simulink model "task_2_sim"  (R2023a)
settings: Solver=VariableStepAuto  StartTime=0.0  StopTime=15  MaxStep=1e-4  RelTol=1e-4
undefined symbols (not defined in the file): A_b, B_b, C_b, D, G, G_g, iQ, K, Kf, Kg, L, w_g0, wfx_0, Y, Y_g
settings Model: Creator=user  LastModifiedBy=user

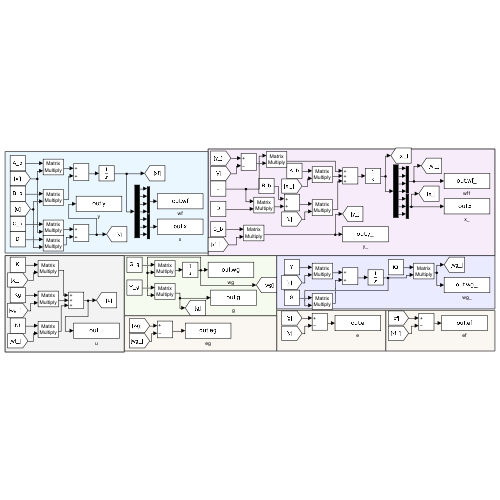
[thumbnail: Simulink's stored preview of the top-level diagram]
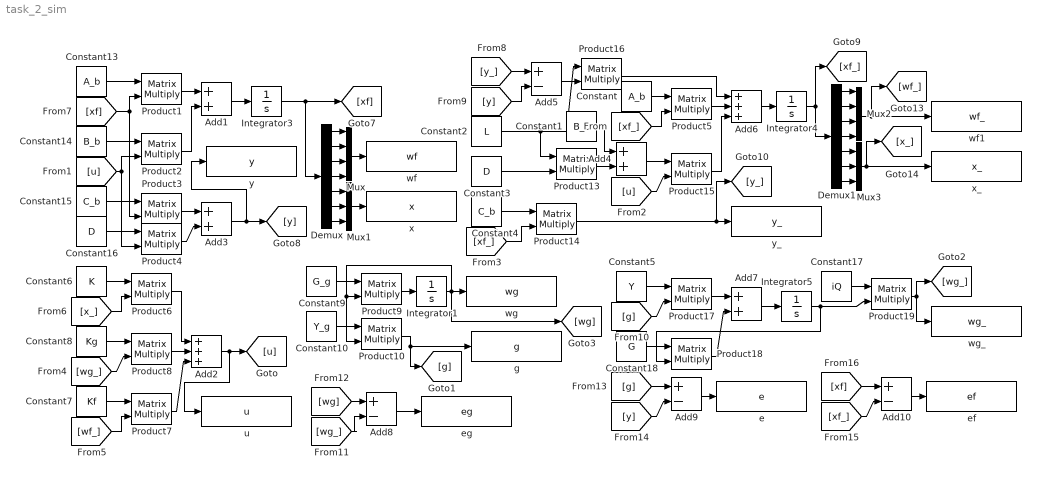
== system task_2_sim ==
  Add{1,3..4,7} (4 alike) : Sum
  Add{5,8..10} (4 alike) : Sum  Inputs=+-
  Add2 : Sum  Inputs=+++
  Add6 : Sum  Inputs=+++
  Constant : Constant  Value=A_b  VectorParams1D=off
  Constant1 : Constant  Value=B_b  VectorParams1D=off
  Constant10 : Constant  Value=Y_g  VectorParams1D=off
  Constant13 : Constant  Value=A_b  VectorParams1D=off
  Constant14 : Constant  Value=B_b  VectorParams1D=off
  Constant15 : Constant  Value=C_b  VectorParams1D=off
  Constant16 : Constant  Value=D  VectorParams1D=off
  Constant17 : Constant  Value=iQ  VectorParams1D=off
  Constant18 : Constant  Value=G  VectorParams1D=off
  Constant2 : Constant  Value=L  VectorParams1D=off
  Constant3 : Constant  Value=D  VectorParams1D=off
  Constant4 : Constant  Value=C_b  VectorParams1D=off
  Constant5 : Constant  Value=Y  VectorParams1D=off
  Constant6 : Constant  Value=K  VectorParams1D=off
  Constant7 : Constant  Value=Kf  VectorParams1D=off
  Constant8 : Constant  Value=Kg  VectorParams1D=off
  Constant9 : Constant  Value=G_g  VectorParams1D=off
  Demux : Demux  Outputs=7
  Demux1 : Demux  Outputs=7
  Integrator1 : Integrator  InitialCondition=w_g0
  Integrator3 : Integrator  InitialCondition=wfx_0
  Integrator4 : Integrator
  Integrator5 : Integrator
  Mux : Mux
  Mux1 : Mux  Inputs=3
  Mux2 : Mux
  Mux3 : Mux  Inputs=3
  Product{1..10,13..19} (17 alike) : Product  Multiplication=Matrix(*)
  e : ToWorkspace  VariableName=e  SaveFormat=Timeseries  SampleTime=-1
  ef : ToWorkspace  VariableName=ef  SaveFormat=Timeseries  SampleTime=-1
  eg : ToWorkspace  VariableName=eg  SaveFormat=Timeseries  SampleTime=-1
  g : ToWorkspace  VariableName=g  SaveFormat=Timeseries  SampleTime=-1
  u : ToWorkspace  VariableName=u  SaveFormat=Timeseries  SampleTime=-1
  wf : ToWorkspace  VariableName=wf  SaveFormat=Timeseries  SampleTime=-1
  wf1 : ToWorkspace  VariableName=wf_  SaveFormat=Timeseries  SampleTime=-1
  wg : ToWorkspace  VariableName=wg  SaveFormat=Timeseries  SampleTime=-1
  wg_ : ToWorkspace  VariableName=wg_  SaveFormat=Timeseries  SampleTime=-1
  x : ToWorkspace  VariableName=x  SaveFormat=Timeseries  SampleTime=-1
  x_ : ToWorkspace  VariableName=x_  SaveFormat=Timeseries  SampleTime=-1
  y : ToWorkspace  VariableName=y  SaveFormat=Timeseries  SampleTime=-1
  y_ : ToWorkspace  VariableName=y_  SaveFormat=Timeseries  SampleTime=-1
  wires:
  Constant6/1 -> Product6/1
  [x_] -> Product6/2
  Constant8/1 -> Product8/1
  [wg_] -> Product8/2
  Constant7/1 -> Product7/1
  [wf_] -> Product7/2
  Product8/1 -> Add2/2
  Product6/1 -> Add2/1
  Product7/1 -> Add2/3
  Add2/1 -> [u], u/1
  Constant9/1 -> Product9/1
  Product9/1 -> Integrator1/1
  Constant10/1 -> Product10/1
  Integrator1/1 -> [wg], Product10/2, Product9/2, wg/1
  Product10/1 -> g/1, [g]
  Constant13/1 -> Product1/1
  [xf] -> Product3/2, Product1/2
  Constant14/1 -> Product2/1
  [u] -> Product4/2, Product2/2
  Constant16/1 -> Product4/1
  Constant15/1 -> Product3/1
  Product1/1 -> Add1/1
  Product2/1 -> Add1/2
  Product3/1 -> Add3/1
  Product4/1 -> Add3/2
  Add1/1 -> Integrator3/1
  Integrator3/1 -> [xf], Demux/1
  Add3/1 -> [y], y/1
  Constant/1 -> Product5/1
  [xf_] -> Product5/2
  Constant2/1 -> Product13/1, Product16/1
  Constant3/1 -> Product13/2
  Constant4/1 -> Product14/1
  [xf_] -> Product14/2
  Product14/1 -> y_/1, [y_]
  Product13/1 -> Add4/2
  Constant1/1 -> Add4/1
  Add4/1 -> Product15/1
  [u] -> Product15/2
  [y_] -> Add5/1
  [y] -> Add5/2
  Add5/1 -> Product16/2
  Product5/1 -> Add6/2
  Product16/1 -> Add6/1
  Product15/1 -> Add6/3
  Add6/1 -> Integrator4/1
  Constant5/1 -> Product17/1
  [g] -> Product17/2
  Product17/1 -> Add7/1
  Add7/1 -> Integrator5/1
  Constant18/1 -> Product18/1
  Integrator5/1 -> Product19/2, Product18/2
  Product18/1 -> Add7/2
  Constant17/1 -> Product19/1
  Product19/1 -> wg_/1, [wg_]
  Demux/1 -> Mux/1
  Demux/2 -> Mux/2
  Demux/3 -> Mux/3
  Demux/4 -> Mux/4
  Mux/1 -> wf/1
  Demux/6 -> Mux1/2
  Demux/5 -> Mux1/1
  Demux/7 -> Mux1/3
  Mux1/1 -> x/1
  Demux1/5 -> Mux3/1
  Mux3/1 -> x_/1, [x_]
  Demux1/4 -> Mux2/4
  Demux1/7 -> Mux3/3
  Demux1/3 -> Mux2/3
  Demux1/2 -> Mux2/2
  Demux1/6 -> Mux3/2
  Mux2/1 -> wf1/1, [wf_]
  Demux1/1 -> Mux2/1
  Integrator4/1 -> [xf_], Demux1/1
  [wg] -> Add8/1
  [wg_] -> Add8/2
  Add8/1 -> eg/1
  [g] -> Add9/1
  [y] -> Add9/2
  Add9/1 -> e/1
  [xf_] -> Add10/2
  [xf] -> Add10/1
  Add10/1 -> ef/1
